simulink model "3R_PD_Regulation_Control"  (R2026a)
settings: Solver=VariableStepAuto
undefined symbols (not defined in the file): X, Y, Z
libraries: nesl_utility x37, sm_lib x29
settings Model: Creator=Bosey  LastModifiedBy=Bosey

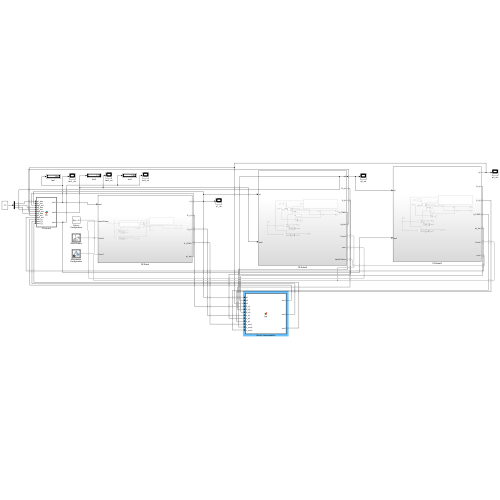
[thumbnail: Simulink's stored preview of the top-level diagram]
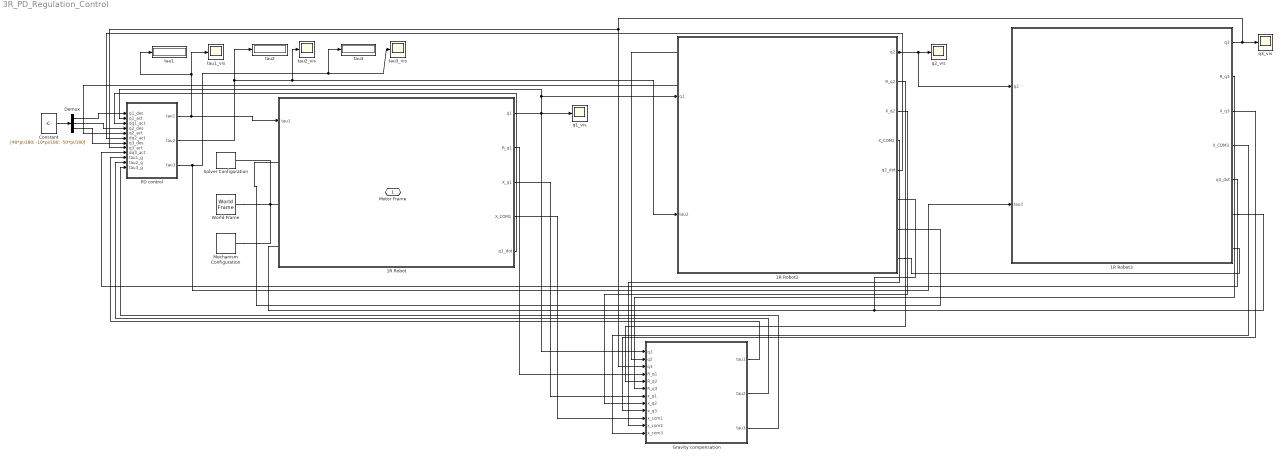
== system 3R_PD_Regulation_Control ==
  1R Robot : Subsystem
  1R Robot2 : Subsystem
  1R Robot3 : Subsystem
  Constant : Constant  Value=[40*pi/180; -10*pi/180; -50*pi/180]
  Demux : Demux  Outputs=3
  Gravity compensation : MATLAB Function  TreatAsAtomicUnit=on
  Mechanism Configuration : sm_lib/Utilities/Mechanism Configuration  UniformGravity=Constant  GravityVector=[0 0 -9.80665]  GravityVectorUnits=m/s^2  LinearizationDelta=0.001  JointModeTransitionNonlinearIterations=2
  PD control : MATLAB Function  TreatAsAtomicUnit=on
  Solver Configuration : nesl_utility/Solver Configuration  PhysicalDomain=network_engine_domain  SubClassName=solver  LeftPortType=input  RightPortType=generic  Tones=[]  Harmonics=[]  SimulateNoise=off  Profile=off  UseLocalSampling=off  EnableSwitchedLinearOptims=on  FrequencyDomain=off  UseCCode=off  RelTol=0.001  AbsTol=1e-06  MinStep=1e-09  ToWorkspace=off  RevertToSquareIcSolve=off  NumHomotopyIterations=100  PhasorMode=off  PhasorModeNumHarmonics=1  ConsistencySolver=NEWTON_XTOL_AFTER_FTOL  CanonicalOrdering=UNORDERED  OptimizeIntermediates=UNOPTIMIZED  IndexReductionMethod=DerivativeReplacement  DoDC=off  ResidualTolerance=1e-09  ConsistencyTolSource=GLOBAL  ConsistencyAbsTol=0.001  ConsistencyRelTol=0.001  ConsistencyTolFactor=0.001  UseLocalSolver=off  LocalSolverChoice=NE_BACKWARD_EULER_ADVANCER  ResolveIndetEquations=on  FunctionEvalNumThread=1  LocalSolverSampleTime=0.001  DoFixedCost=off  MaxNonlinIter=3  MaxModeIter=2  ComputeImpulses=off  ImpulseIterations=2  LinearAlgebra=Sparse  LinearAlgebraNumThread=0  EquationFormulation=NE_TIME_EF  DelaysMemoryBudget=1024  AutomaticFiltering=on  FilteringTimeConstant=0.001  PartitionStorageMethod=AS_NEEDED  PartitionMemoryBudget=1024  PartitionMethod=FAST  MultibodyUseLocalSolver=off  MultibodyLocalSolverChoice=ODE1  MultibodyLocalSolverSampleTime=0.001
  World Frame : sm_lib/Frames and Transforms/World Frame
  q1_vis : Scope
      settings: ActiveDisplayYMinimum=0.2274863959797675  ActiveDisplayYMaximum=1.3862172206154479
  q2_vis : Scope
      settings: ActiveDisplayYMinimum=-0.21838931601721817  ActiveDisplayYMaximum=0.20349654350607727  DataLoggingVariableName=ScopeData4
  q3_vis : Scope
      settings: ActiveDisplayYMinimum=-0.90239032801862251  ActiveDisplayYMaximum=-0.64728032168659821  DataLoggingVariableName=ScopeData11
  tau1 : Display
  tau1_vis : Scope
      settings: ActiveDisplayYMinimum=-1  ActiveDisplayYMaximum=1  DataLoggingVariableName=ScopeData8
  tau2 : Display
  tau2_vis : Scope
      settings: DataLoggingVariableName=ScopeData9
  tau3 : Display
  tau3_vis : Scope
      settings: DataLoggingVariableName=ScopeData10
  Motor Frame : PMIOPort  Side=Left
  wires:
  1R Robot2/1(q2) -> Gravity compensation/2(q2), PD control/5(q2_act), 1R Robot3/1(q2), q2_vis/1
  1R Robot/1(q1) -> Gravity compensation/1(q1), PD control/2(q1_act), 1R Robot2/1(q1), q1_vis/1
  1R Robot/3(X_q1) -> Gravity compensation/7(x_q1)
  1R Robot2/3(X_q2) -> Gravity compensation/8(x_q2)
  1R Robot3/4(X_COM3) -> Gravity compensation/12(x_com3)
  1R Robot3/3(X_q3) -> Gravity compensation/9(x_q3)
  1R Robot2/4(X_COM2) -> Gravity compensation/11(x_com2)
  1R Robot3/1(q3) -> q3_vis/1, PD control/8(q3_act), Gravity compensation/3(q3)
  1R Robot/4(X_COM1) -> Gravity compensation/10(x_com1)
  PD control/1(tau1) -> tau1_vis/1, tau1/1, 1R Robot/1(tau1)
  PD control/2(tau2) -> tau2/1, 1R Robot2/2(tau2), tau2_vis/1
  PD control/3(tau3) -> tau3_vis/1, tau3/1, 1R Robot3/2(tau3)
  1R Robot/5(q1_dot) -> PD control/3(dq1_act)
  1R Robot2/5(q2_dot) -> PD control/6(dq2_act)
  1R Robot3/5(q3_dot) -> PD control/9(dq3_act)
  1R Robot/2(R_q1) -> Gravity compensation/4(R_q1)
  1R Robot2/2(R_q2) -> Gravity compensation/5(R_q2)
  Gravity compensation/1(tau1) -> PD control/10(tau1_g)
  Gravity compensation/2(tau2) -> PD control/11(tau2_g)
  1R Robot3/2(R_q3) -> Gravity compensation/6(R_q3)
  Gravity compensation/3(tau3) -> PD control/12(tau3_g)
  Constant/1 -> Demux/1
  Demux/1 -> PD control/1(q1_des)
  Demux/2 -> PD control/4(q2_des)
  Demux/3 -> PD control/7(q3_des)
  connections:
  Solver Configuration/RConn1 -- Mechanism Configuration/RConn1 -- World Frame/RConn1 -- 1R Robot/LConn2
  1R Robot2/RConn1 -- 1R Robot/LConn3 -- 1R Robot3/RConn1
  1R Robot/LConn1 -- 1R Robot2/RConn2
  1R Robot2/RConn3 -- 1R Robot3/RConn2

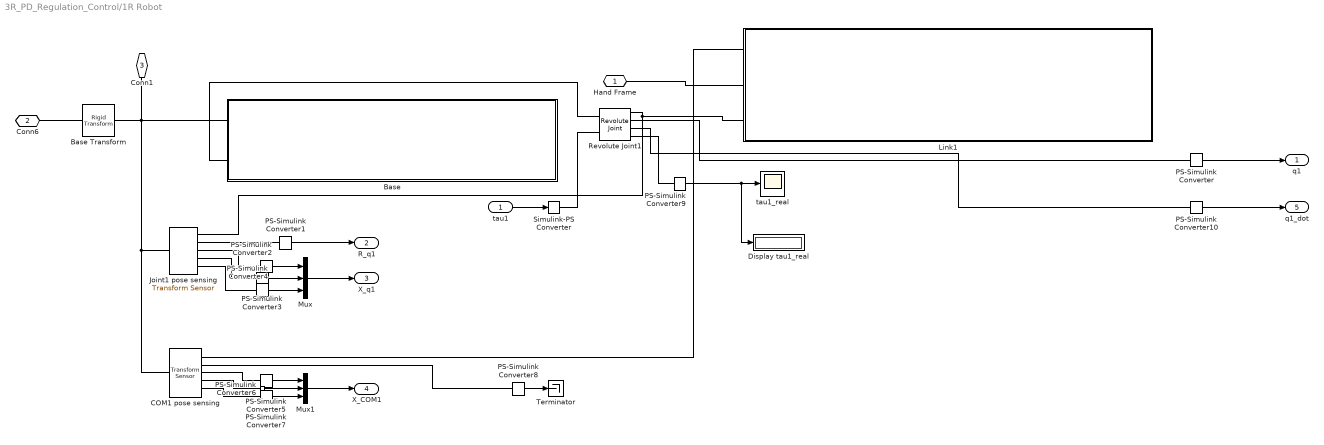
== system 3R_PD_Regulation_Control/1R Robot ==
  tau1 : Inport
  Base : Subsystem
  Base Transform : sm_lib/Frames and Transforms/Rigid Transform  RotationMethod=RotationMatrix  FollAlignAxisA=+Z  BaseAlignAxisA=-Y  FollAlignAxisB=+X  BaseAlignAxisB=+X  RotationStandardAxis=+X  RotationAngle=90  RotationAngleUnits=deg  RotationArbitraryAxis=[0 0 1]  RotationSequenceAxes=BaseAxes  RotationSequence=XYZ  RotationSequenceAngles=[90 0 0]  RotationSequenceAnglesUnits=deg  RotationMatrix=[1 0 0; 0 0 -1; 0 1 0]  Quaternion=[1 0 0 0]  TranslationMethod=None  TranslationCartesianOffset=[0 0 0]  TranslationCartesianOffsetUnits=m  TranslationStandardAxis=+Z  TranslationStandardOffset=0  TranslationStandardOffsetUnits=m  TranslationROffset=0  TranslationROffsetUnits=m  TranslationThetaOffset=0  TranslationThetaOffsetUnits=deg  TranslationZOffset=0  TranslationZOffsetUnits=m
  COM1 pose sensing : sm_lib/Frames and Transforms/Transform Sensor  MeasurementFrame=Base  RotationSequence=XYX  SenseAngle=off  SenseAxis=off  SenseQ=off  SenseR=on  SenseRotationSequence=off  SenseOmegaX=off  SenseOmegaY=off  SenseOmegaZ=off  SenseOmega=off  SenseQDot=off  SenseRDot=off  SenseRotationSequenceDot=off  SenseAlphaX=off  SenseAlphaY=off  SenseAlphaZ=off  SenseAlpha=off  SenseQDDot=off  SenseRDDot=off  SenseX=on  SenseY=on  SenseZ=on  SenseXYZ=off  SenseRad=off  SenseAzim=off  SenseDist=off  SenseInc=off  SenseXDot=off  SenseYDot=off  SenseZDot=off  SenseXYZDot=off  SenseRadDot=off  SenseAzimDot=off  SenseDistDot=off  SenseIncDot=off  SenseXDDot=off  SenseYDDot=off  SenseZDDot=off  SenseXYZDDot=off  SenseRadDDot=off  SenseAzimDDot=off  SenseDistDDot=off  SenseIncDDot=off
  Display tau1_real : Display
  Joint1 pose sensing : sm_lib/Frames and Transforms/Transform Sensor  MeasurementFrame=Base  RotationSequence=XYX  SenseAngle=off  SenseAxis=off  SenseQ=off  SenseR=on  SenseRotationSequence=off  SenseOmegaX=off  SenseOmegaY=off  SenseOmegaZ=off  SenseOmega=off  SenseQDot=off  SenseRDot=off  SenseRotationSequenceDot=off  SenseAlphaX=off  SenseAlphaY=off  SenseAlphaZ=off  SenseAlpha=off  SenseQDDot=off  SenseRDDot=off  SenseX=on  SenseY=on  SenseZ=on  SenseXYZ=off  SenseRad=off  SenseAzim=off  SenseDist=off  SenseInc=off  SenseXDot=off  SenseYDot=off  SenseZDot=off  SenseXYZDot=off  SenseRadDot=off  SenseAzimDot=off  SenseDistDot=off  SenseIncDot=off  SenseXDDot=off  SenseYDDot=off  SenseZDDot=off  SenseXYZDDot=off  SenseRadDDot=off  SenseAzimDDot=off  SenseDistDDot=off  SenseIncDDot=off
  Link1 : Subsystem
  Mux : Mux  Inputs=3
  Mux1 : Mux  Inputs=3
  PS-Simulink Converter{,1..10} (11 alike) : nesl_utility/PS-Simulink Converter  PhysicalDomain=network_engine_domain  SubClassName=ps_output  LeftPortType=input  RightPortType=output  PseudoPeriodic=off  Frequencies=[]  VectorFormat=inherit  Unit=inherit  AffineConversion=off
  Revolute Joint1 : sm_lib/Joints/Revolute Joint  JointMode=Normal  CompositeWrenchDir=FollowerOnBase  CompositeWrenchFrame=BaseFrame  SenseConstraintForce=off  SenseConstraintTorque=off  SenseTotalForce=off  SenseTotalTorque=off  PositionTargetSpecify=on  PositionTargetPriority=High  PositionTargetValue=10  PositionTargetValueUnits=deg  VelocityTargetSpecify=off  VelocityTargetPriority=High  VelocityTargetValue=0  VelocityTargetValueUnits=deg/s  EquilibriumPosition=0  EquilibriumPositionUnits=deg  SpringStiffness=0  SpringStiffnessUnits=N*m/deg  DampingCoefficient=0  DampingCoefficientUnits=N*m/(deg/s)  LowerLimitSpecify=off  LowerLimitBound=-90  LowerLimitBoundUnits=deg  LowerLimitStiffness=1e4  LowerLimitStiffnessUnits=N*m/deg  LowerLimitDamping=10  LowerLimitDampingUnits=N*m/(deg/s)  LowerLimitTransitionRegionWidth=0.1  LowerLimitTransitionRegionWidthUnits=deg  UpperLimitSpecify=off  UpperLimitBound=90  UpperLimitBoundUnits=deg  UpperLimitStiffness=1e4  UpperLimitStiffnessUnits=N*m/deg  UpperLimitDamping=10  UpperLimitDampingUnits=N*m/(deg/s)  UpperLimitTransitionRegionWidth=0.1  UpperLimitTransitionRegionWidthUnits=deg  TorqueActuationMode=InputTorque  MotionActuationMode=ComputedMotion  SensePosition=on  SenseVelocity=on  SenseAcceleration=off  SenseTorqueForce=on  SenseLowerLimitTorqueForce=off  SenseUpperLimitTorqueForce=off
  Simulink-PS Converter : nesl_utility/Simulink-PS Converter  PhysicalDomain=network_engine_domain  SubClassName=ps_input  LeftPortType=input  RightPortType=output  PseudoPeriodic=off  Frequencies=[]  NoiseDistribution=none  NoiseParameters=[]  Unit=1  AffineConversion=off  FilteringAndDerivatives=provide  SimscapeFilterOrder=1  InputFilterTimeConstant=0.001  UdotUserProvided=0
  Terminator : Terminator
  tau1_real : Scope
      settings: ActiveDisplayYMinimum=-1  ActiveDisplayYMaximum=1
  Hand Frame : PMIOPort  Side=Left
  Conn6 : PMIOPort  Port=2  Side=Left
  Conn1 : PMIOPort  Port=3  Side=Left
  q1 : Outport
  R_q1 : Outport  Port=2
  X_q1 : Outport  Port=3
  X_COM1 : Outport  Port=4
  q1_dot : Outport  Port=5
  wires:
  PS-Simulink Converter/1 -> q1/1
  tau1/1 -> Simulink-PS Converter/1
  PS-Simulink Converter1/1 -> R_q1/1
  PS-Simulink Converter2/1 -> Mux/1
  PS-Simulink Converter3/1 -> Mux/2
  PS-Simulink Converter4/1 -> Mux/3
  Mux/1 -> X_q1/1
  PS-Simulink Converter7/1 -> Mux1/3
  PS-Simulink Converter6/1 -> Mux1/2
  PS-Simulink Converter5/1 -> Mux1/1
  Mux1/1 -> X_COM1/1
  PS-Simulink Converter8/1 -> Terminator/1
  PS-Simulink Converter9/1 -> Display tau1_real/1, tau1_real/1
  PS-Simulink Converter10/1 -> q1_dot/1
  connections:
  Conn1/RConn1 -- Base/LConn1 -- Base Transform/RConn1 -- COM1 pose sensing/LConn1 -- Joint1 pose sensing/LConn1
  Base/LConn2 -- Revolute Joint1/LConn1
  Link1/LConn3 -- Joint1 pose sensing/RConn1 -- Revolute Joint1/RConn1
  COM1 pose sensing/RConn1 -- Link1/LConn1
  Revolute Joint1/RConn2 -- PS-Simulink Converter/LConn1
  Simulink-PS Converter/RConn1 -- Revolute Joint1/LConn2
  Joint1 pose sensing/RConn2 -- PS-Simulink Converter1/LConn1
  COM1 pose sensing/RConn3 -- PS-Simulink Converter5/LConn1
  COM1 pose sensing/RConn4 -- PS-Simulink Converter6/LConn1
  COM1 pose sensing/RConn5 -- PS-Simulink Converter7/LConn1
  COM1 pose sensing/RConn2 -- PS-Simulink Converter8/LConn1
  PS-Simulink Converter2/LConn1 -- Joint1 pose sensing/RConn3
  Joint1 pose sensing/RConn5 -- PS-Simulink Converter4/LConn1
  Joint1 pose sensing/RConn4 -- PS-Simulink Converter3/LConn1
  Hand Frame/RConn1 -- Link1/LConn2
  Base Transform/LConn1 -- Conn6/RConn1
  PS-Simulink Converter9/LConn1 -- Revolute Joint1/RConn4
  PS-Simulink Converter10/LConn1 -- Revolute Joint1/RConn3

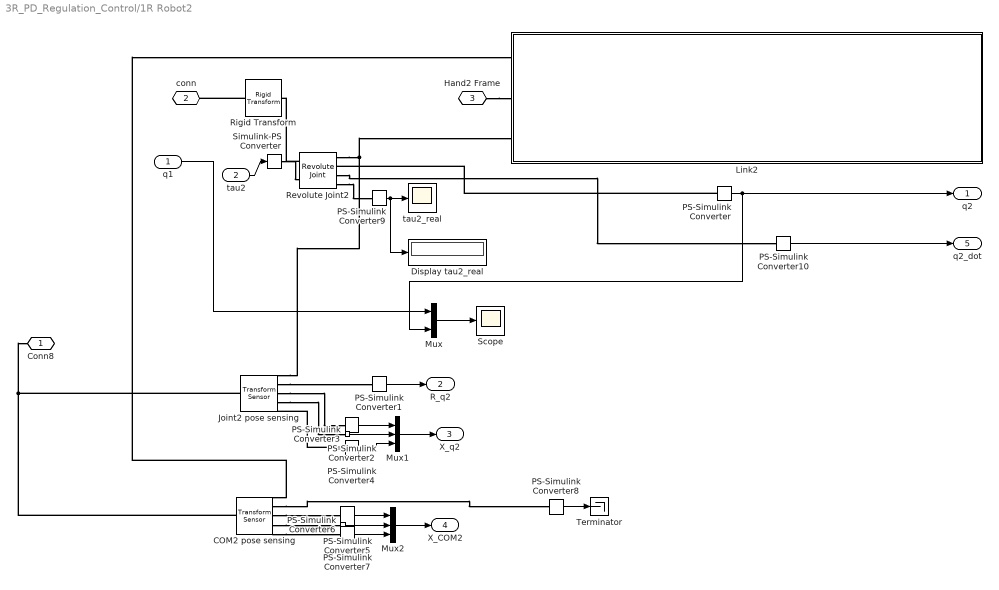
== system 3R_PD_Regulation_Control/1R Robot2 ==
  q1 : Inport
  tau2 : Inport  Port=2
  COM2 pose sensing : sm_lib/Frames and Transforms/Transform Sensor  MeasurementFrame=Base  RotationSequence=XYX  SenseAngle=off  SenseAxis=off  SenseQ=off  SenseR=on  SenseRotationSequence=off  SenseOmegaX=off  SenseOmegaY=off  SenseOmegaZ=off  SenseOmega=off  SenseQDot=off  SenseRDot=off  SenseRotationSequenceDot=off  SenseAlphaX=off  SenseAlphaY=off  SenseAlphaZ=off  SenseAlpha=off  SenseQDDot=off  SenseRDDot=off  SenseX=on  SenseY=on  SenseZ=on  SenseXYZ=off  SenseRad=off  SenseAzim=off  SenseDist=off  SenseInc=off  SenseXDot=off  SenseYDot=off  SenseZDot=off  SenseXYZDot=off  SenseRadDot=off  SenseAzimDot=off  SenseDistDot=off  SenseIncDot=off  SenseXDDot=off  SenseYDDot=off  SenseZDDot=off  SenseXYZDDot=off  SenseRadDDot=off  SenseAzimDDot=off  SenseDistDDot=off  SenseIncDDot=off
  Display tau2_real : Display
  Joint2 pose sensing : sm_lib/Frames and Transforms/Transform Sensor  MeasurementFrame=Base  RotationSequence=XYX  SenseAngle=off  SenseAxis=off  SenseQ=off  SenseR=on  SenseRotationSequence=off  SenseOmegaX=off  SenseOmegaY=off  SenseOmegaZ=off  SenseOmega=off  SenseQDot=off  SenseRDot=off  SenseRotationSequenceDot=off  SenseAlphaX=off  SenseAlphaY=off  SenseAlphaZ=off  SenseAlpha=off  SenseQDDot=off  SenseRDDot=off  SenseX=on  SenseY=on  SenseZ=on  SenseXYZ=off  SenseRad=off  SenseAzim=off  SenseDist=off  SenseInc=off  SenseXDot=off  SenseYDot=off  SenseZDot=off  SenseXYZDot=off  SenseRadDot=off  SenseAzimDot=off  SenseDistDot=off  SenseIncDot=off  SenseXDDot=off  SenseYDDot=off  SenseZDDot=off  SenseXYZDDot=off  SenseRadDDot=off  SenseAzimDDot=off  SenseDistDDot=off  SenseIncDDot=off
  Link2 : Subsystem
  Mux : Mux  Inputs=2
  Mux1 : Mux  Inputs=3
  Mux2 : Mux  Inputs=3
  PS-Simulink Converter{,1..10} (11 alike) : nesl_utility/PS-Simulink Converter  PhysicalDomain=network_engine_domain  SubClassName=ps_output  LeftPortType=input  RightPortType=output  PseudoPeriodic=off  Frequencies=[]  VectorFormat=inherit  Unit=inherit  AffineConversion=off
  Revolute Joint2 : sm_lib/Joints/Revolute Joint  JointMode=Normal  CompositeWrenchDir=FollowerOnBase  CompositeWrenchFrame=BaseFrame  SenseConstraintForce=off  SenseConstraintTorque=off  SenseTotalForce=off  SenseTotalTorque=off  PositionTargetSpecify=on  PositionTargetPriority=High  PositionTargetValue=20  PositionTargetValueUnits=deg  VelocityTargetSpecify=off  VelocityTargetPriority=High  VelocityTargetValue=0  VelocityTargetValueUnits=deg/s  EquilibriumPosition=0  EquilibriumPositionUnits=deg  SpringStiffness=0  SpringStiffnessUnits=N*m/deg  DampingCoefficient=0  DampingCoefficientUnits=N*m/(deg/s)  LowerLimitSpecify=off  LowerLimitBound=-90  LowerLimitBoundUnits=deg  LowerLimitStiffness=1e4  LowerLimitStiffnessUnits=N*m/deg  LowerLimitDamping=10  LowerLimitDampingUnits=N*m/(deg/s)  LowerLimitTransitionRegionWidth=0.1  LowerLimitTransitionRegionWidthUnits=deg  UpperLimitSpecify=off  UpperLimitBound=90  UpperLimitBoundUnits=deg  UpperLimitStiffness=1e4  UpperLimitStiffnessUnits=N*m/deg  UpperLimitDamping=10  UpperLimitDampingUnits=N*m/(deg/s)  UpperLimitTransitionRegionWidth=0.1  UpperLimitTransitionRegionWidthUnits=deg  TorqueActuationMode=InputTorque  MotionActuationMode=ComputedMotion  SensePosition=on  SenseVelocity=on  SenseAcceleration=off  SenseTorqueForce=on  SenseLowerLimitTorqueForce=off  SenseUpperLimitTorqueForce=off
  Rigid Transform : sm_lib/Frames and Transforms/Rigid Transform  RotationMethod=None  FollAlignAxisA=+X  BaseAlignAxisA=+Y  FollAlignAxisB=+Y  BaseAlignAxisB=+Z  RotationStandardAxis=+Z  RotationAngle=90  RotationAngleUnits=deg  RotationArbitraryAxis=[0 0 1]  RotationSequenceAxes=BaseAxes  RotationSequence=XYZ  RotationSequenceAngles=[-90 0 -90]  RotationSequenceAnglesUnits=deg  RotationMatrix=[1 0 0;0 1 0;0 0 1]  Quaternion=[1 0 0 0]  TranslationMethod=None  TranslationCartesianOffset=[0 0 0]  TranslationCartesianOffsetUnits=m  TranslationStandardAxis=+X  TranslationStandardOffset=0.2  TranslationStandardOffsetUnits=m  TranslationROffset=0  TranslationROffsetUnits=m  TranslationThetaOffset=0  TranslationThetaOffsetUnits=deg  TranslationZOffset=0  TranslationZOffsetUnits=m
  Scope : Scope
      settings: ActiveDisplayYMinimum=-3.9555769196396309  ActiveDisplayYMaximum=1.3121731726237904
  Simulink-PS Converter : nesl_utility/Simulink-PS Converter  PhysicalDomain=network_engine_domain  SubClassName=ps_input  LeftPortType=input  RightPortType=output  PseudoPeriodic=off  Frequencies=[]  NoiseDistribution=none  NoiseParameters=[]  Unit=1  AffineConversion=off  FilteringAndDerivatives=provide  SimscapeFilterOrder=1  InputFilterTimeConstant=0.001  UdotUserProvided=0
  Terminator : Terminator
  tau2_real : Scope
      settings: ActiveDisplayYMinimum=-1  ActiveDisplayYMaximum=1  DataLoggingVariableName=ScopeData7
  Conn8 : PMIOPort  Side=Right
  conn : PMIOPort  Port=2  Side=Right
  Hand2 Frame : PMIOPort  Port=3  Side=Right
  q2 : Outport
  R_q2 : Outport  Port=2
  X_q2 : Outport  Port=3
  X_COM2 : Outport  Port=4
  q2_dot : Outport  Port=5
  wires:
  PS-Simulink Converter8/1 -> Terminator/1
  PS-Simulink Converter4/1 -> Mux1/3
  Mux/1 -> Scope/1
  Mux1/1 -> X_q2/1
  PS-Simulink Converter2/1 -> Mux1/1
  PS-Simulink Converter7/1 -> Mux2/3
  PS-Simulink Converter3/1 -> Mux1/2
  PS-Simulink Converter1/1 -> R_q2/1
  PS-Simulink Converter6/1 -> Mux2/2
  Mux2/1 -> X_COM2/1
  PS-Simulink Converter5/1 -> Mux2/1
  q1/1 -> Mux/1
  PS-Simulink Converter9/1 -> Display tau2_real/1, tau2_real/1
  tau2/1 -> Simulink-PS Converter/1
  PS-Simulink Converter/1 -> Mux/2, q2/1
  PS-Simulink Converter10/1 -> q2_dot/1
  connections:
  PS-Simulink Converter4/LConn1 -- Joint2 pose sensing/RConn5
  COM2 pose sensing/RConn1 -- Link2/LConn1
  Revolute Joint2/RConn1 -- Link2/LConn3 -- Joint2 pose sensing/RConn1
  PS-Simulink Converter/LConn1 -- Revolute Joint2/RConn2
  Joint2 pose sensing/RConn3 -- PS-Simulink Converter2/LConn1
  Joint2 pose sensing/LConn1 -- COM2 pose sensing/LConn1 -- Conn8/RConn1
  Joint2 pose sensing/RConn2 -- PS-Simulink Converter1/LConn1
  COM2 pose sensing/RConn5 -- PS-Simulink Converter7/LConn1
  COM2 pose sensing/RConn4 -- PS-Simulink Converter6/LConn1
  COM2 pose sensing/RConn3 -- PS-Simulink Converter5/LConn1
  COM2 pose sensing/RConn2 -- PS-Simulink Converter8/LConn1
  Joint2 pose sensing/RConn4 -- PS-Simulink Converter3/LConn1
  Rigid Transform/LConn1 -- conn/RConn1
  Revolute Joint2/LConn1 -- Rigid Transform/RConn1
  Revolute Joint2/RConn4 -- PS-Simulink Converter9/LConn1
  Revolute Joint2/RConn3 -- PS-Simulink Converter10/LConn1
  Simulink-PS Converter/RConn1 -- Revolute Joint2/LConn2
  Hand2 Frame/RConn1 -- Link2/LConn2

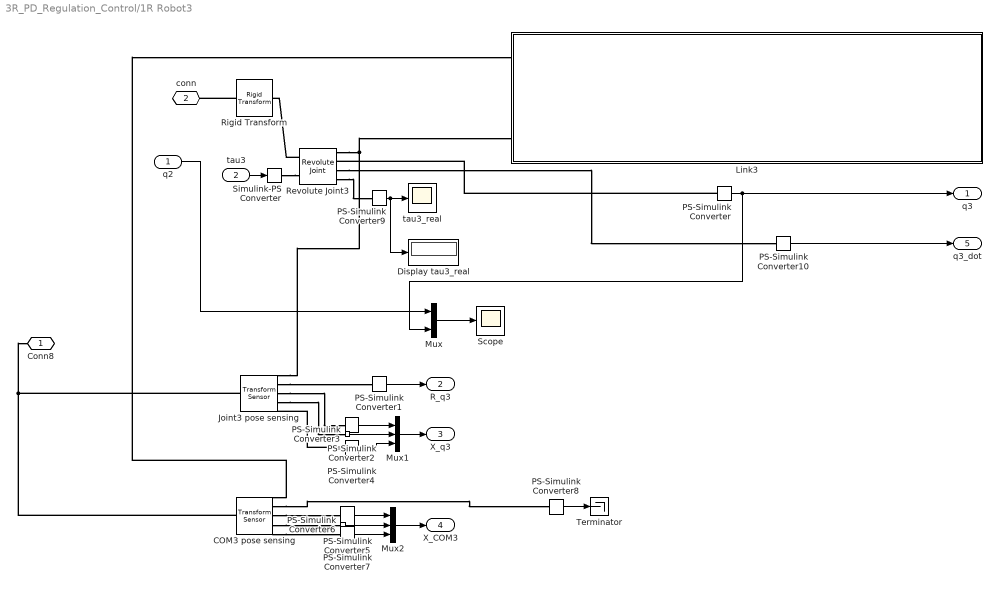
== system 3R_PD_Regulation_Control/1R Robot3 ==
  q2 : Inport
  tau3 : Inport  Port=2
  COM3 pose sensing : sm_lib/Frames and Transforms/Transform Sensor  MeasurementFrame=Base  RotationSequence=XYX  SenseAngle=off  SenseAxis=off  SenseQ=off  SenseR=on  SenseRotationSequence=off  SenseOmegaX=off  SenseOmegaY=off  SenseOmegaZ=off  SenseOmega=off  SenseQDot=off  SenseRDot=off  SenseRotationSequenceDot=off  SenseAlphaX=off  SenseAlphaY=off  SenseAlphaZ=off  SenseAlpha=off  SenseQDDot=off  SenseRDDot=off  SenseX=on  SenseY=on  SenseZ=on  SenseXYZ=off  SenseRad=off  SenseAzim=off  SenseDist=off  SenseInc=off  SenseXDot=off  SenseYDot=off  SenseZDot=off  SenseXYZDot=off  SenseRadDot=off  SenseAzimDot=off  SenseDistDot=off  SenseIncDot=off  SenseXDDot=off  SenseYDDot=off  SenseZDDot=off  SenseXYZDDot=off  SenseRadDDot=off  SenseAzimDDot=off  SenseDistDDot=off  SenseIncDDot=off
  Display tau3_real : Display
  Joint3 pose sensing : sm_lib/Frames and Transforms/Transform Sensor  MeasurementFrame=Base  RotationSequence=XYX  SenseAngle=off  SenseAxis=off  SenseQ=off  SenseR=on  SenseRotationSequence=off  SenseOmegaX=off  SenseOmegaY=off  SenseOmegaZ=off  SenseOmega=off  SenseQDot=off  SenseRDot=off  SenseRotationSequenceDot=off  SenseAlphaX=off  SenseAlphaY=off  SenseAlphaZ=off  SenseAlpha=off  SenseQDDot=off  SenseRDDot=off  SenseX=on  SenseY=on  SenseZ=on  SenseXYZ=off  SenseRad=off  SenseAzim=off  SenseDist=off  SenseInc=off  SenseXDot=off  SenseYDot=off  SenseZDot=off  SenseXYZDot=off  SenseRadDot=off  SenseAzimDot=off  SenseDistDot=off  SenseIncDot=off  SenseXDDot=off  SenseYDDot=off  SenseZDDot=off  SenseXYZDDot=off  SenseRadDDot=off  SenseAzimDDot=off  SenseDistDDot=off  SenseIncDDot=off
  Link3 : Subsystem
  Mux : Mux  Inputs=2
  Mux1 : Mux  Inputs=3
  Mux2 : Mux  Inputs=3
  PS-Simulink Converter{,1..10} (11 alike) : nesl_utility/PS-Simulink Converter  PhysicalDomain=network_engine_domain  SubClassName=ps_output  LeftPortType=input  RightPortType=output  PseudoPeriodic=off  Frequencies=[]  VectorFormat=inherit  Unit=inherit  AffineConversion=off
  Revolute Joint3 : sm_lib/Joints/Revolute Joint  JointMode=Normal  CompositeWrenchDir=FollowerOnBase  CompositeWrenchFrame=BaseFrame  SenseConstraintForce=off  SenseConstraintTorque=off  SenseTotalForce=off  SenseTotalTorque=off  PositionTargetSpecify=on  PositionTargetPriority=High  PositionTargetValue=-30  PositionTargetValueUnits=deg  VelocityTargetSpecify=off  VelocityTargetPriority=High  VelocityTargetValue=0  VelocityTargetValueUnits=deg/s  EquilibriumPosition=0  EquilibriumPositionUnits=deg  SpringStiffness=0  SpringStiffnessUnits=N*m/deg  DampingCoefficient=0  DampingCoefficientUnits=N*m/(deg/s)  LowerLimitSpecify=off  LowerLimitBound=-90  LowerLimitBoundUnits=deg  LowerLimitStiffness=1e4  LowerLimitStiffnessUnits=N*m/deg  LowerLimitDamping=10  LowerLimitDampingUnits=N*m/(deg/s)  LowerLimitTransitionRegionWidth=0.1  LowerLimitTransitionRegionWidthUnits=deg  UpperLimitSpecify=off  UpperLimitBound=90  UpperLimitBoundUnits=deg  UpperLimitStiffness=1e4  UpperLimitStiffnessUnits=N*m/deg  UpperLimitDamping=10  UpperLimitDampingUnits=N*m/(deg/s)  UpperLimitTransitionRegionWidth=0.1  UpperLimitTransitionRegionWidthUnits=deg  TorqueActuationMode=InputTorque  MotionActuationMode=ComputedMotion  SensePosition=on  SenseVelocity=on  SenseAcceleration=off  SenseTorqueForce=on  SenseLowerLimitTorqueForce=off  SenseUpperLimitTorqueForce=off
  Rigid Transform : sm_lib/Frames and Transforms/Rigid Transform  RotationMethod=None  FollAlignAxisA=+X  BaseAlignAxisA=+Y  FollAlignAxisB=+Y  BaseAlignAxisB=+Z  RotationStandardAxis=+Z  RotationAngle=90  RotationAngleUnits=deg  RotationArbitraryAxis=[0 0 1]  RotationSequenceAxes=BaseAxes  RotationSequence=XYZ  RotationSequenceAngles=[-90 0 -90]  RotationSequenceAnglesUnits=deg  RotationMatrix=[1 0 0;0 1 0;0 0 1]  Quaternion=[1 0 0 0]  TranslationMethod=None  TranslationCartesianOffset=[0 0 0]  TranslationCartesianOffsetUnits=m  TranslationStandardAxis=+X  TranslationStandardOffset=0.2  TranslationStandardOffsetUnits=m  TranslationROffset=0  TranslationROffsetUnits=m  TranslationThetaOffset=0  TranslationThetaOffsetUnits=deg  TranslationZOffset=0  TranslationZOffsetUnits=m
  Scope : Scope
      settings: ActiveDisplayYMinimum=-3.9555769196396309  ActiveDisplayYMaximum=1.3121731726237904
  Simulink-PS Converter : nesl_utility/Simulink-PS Converter  PhysicalDomain=network_engine_domain  SubClassName=ps_input  LeftPortType=input  RightPortType=output  PseudoPeriodic=off  Frequencies=[]  NoiseDistribution=none  NoiseParameters=[]  Unit=1  AffineConversion=off  FilteringAndDerivatives=provide  SimscapeFilterOrder=1  InputFilterTimeConstant=0.001  UdotUserProvided=0
  Terminator : Terminator
  tau3_real : Scope
      settings: ActiveDisplayYMinimum=0.20752725828747631  ActiveDisplayYMaximum=1.0145136066212581  DataLoggingVariableName=ScopeData7
  Conn8 : PMIOPort  Side=Right
  conn : PMIOPort  Port=2  Side=Right
  q3 : Outport
  R_q3 : Outport  Port=2
  X_q3 : Outport  Port=3
  X_COM3 : Outport  Port=4
  q3_dot : Outport  Port=5
  wires:
  PS-Simulink Converter8/1 -> Terminator/1
  PS-Simulink Converter4/1 -> Mux1/3
  Mux/1 -> Scope/1
  Mux1/1 -> X_q3/1
  PS-Simulink Converter2/1 -> Mux1/1
  PS-Simulink Converter7/1 -> Mux2/3
  PS-Simulink Converter3/1 -> Mux1/2
  PS-Simulink Converter1/1 -> R_q3/1
  PS-Simulink Converter6/1 -> Mux2/2
  Mux2/1 -> X_COM3/1
  PS-Simulink Converter5/1 -> Mux2/1
  q2/1 -> Mux/1
  PS-Simulink Converter9/1 -> Display tau3_real/1, tau3_real/1
  tau3/1 -> Simulink-PS Converter/1
  PS-Simulink Converter/1 -> Mux/2, q3/1
  PS-Simulink Converter10/1 -> q3_dot/1
  connections:
  PS-Simulink Converter4/LConn1 -- Joint3 pose sensing/RConn5
  COM3 pose sensing/RConn1 -- Link3/LConn1
  Revolute Joint3/RConn1 -- Link3/LConn3 -- Joint3 pose sensing/RConn1
  PS-Simulink Converter/LConn1 -- Revolute Joint3/RConn2
  Joint3 pose sensing/RConn3 -- PS-Simulink Converter2/LConn1
  Joint3 pose sensing/LConn1 -- COM3 pose sensing/LConn1 -- Conn8/RConn1
  Joint3 pose sensing/RConn2 -- PS-Simulink Converter1/LConn1
  COM3 pose sensing/RConn5 -- PS-Simulink Converter7/LConn1
  COM3 pose sensing/RConn4 -- PS-Simulink Converter6/LConn1
  COM3 pose sensing/RConn3 -- PS-Simulink Converter5/LConn1
  COM3 pose sensing/RConn2 -- PS-Simulink Converter8/LConn1
  Joint3 pose sensing/RConn4 -- PS-Simulink Converter3/LConn1
  Rigid Transform/LConn1 -- conn/RConn1
  Revolute Joint3/LConn1 -- Rigid Transform/RConn1
  Revolute Joint3/RConn4 -- PS-Simulink Converter9/LConn1
  Revolute Joint3/RConn3 -- PS-Simulink Converter10/LConn1
  Simulink-PS Converter/RConn1 -- Revolute Joint3/LConn2

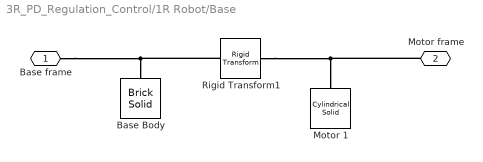
== system 3R_PD_Regulation_Control/1R Robot/Base ==
  "Base Body " : sm_lib/Body Elements/Brick Solid  BrickDimensions=[0.2 0.2 0.02]  BrickDimensionsUnits=m  ExportEntireGeometry=off  InertiaType=CalculateFromGeometry  BasedOnType=Mass  Density=1000  DensityUnits=kg/m^3  Mass=0  MassUnits=kg  CenterOfMass=[0 0 0]  CenterOfMassUnits=m  MomentsOfInertia=[1 1 1]  MomentsOfInertiaUnits=kg*m^2  ProductsOfInertia=[0 0 0]  ProductsOfInertiaUnits=kg*m^2  GraphicType=FromGeometry  MarkerShape=Sphere  MarkerSize=10  GraphicVisPropType=SimpleVisualProperties  GraphicDiffuseColor=[0.502 0.502 0.502]  GraphicOpacity=1.0  GraphicSpecularColor=[0.5 0.5 0.5 1.0]  GraphicAmbientColor=[0.15 0.15 0.15 1.0]  GraphicEmissiveColor=[0.0 0.0 0.0 1.0]  GraphicShininess=75  DoExposeReferenceFrame=on  SerializedFrames=<Frames/>
  Motor 1 : sm_lib/Body Elements/Cylindrical Solid  CylinderRadius=0.02  CylinderRadiusUnits=m  CylinderLength=0.04  CylinderLengthUnits=m  ExportEntireGeometry=off  InertiaType=CalculateFromGeometry  BasedOnType=Mass  Density=1000  DensityUnits=kg/m^3  Mass=0  MassUnits=kg  CenterOfMass=[0 0 0]  CenterOfMassUnits=m  MomentsOfInertia=[1 1 1]  MomentsOfInertiaUnits=kg*m^2  ProductsOfInertia=[0 0 0]  ProductsOfInertiaUnits=kg*m^2  GraphicType=FromGeometry  MarkerShape=Sphere  MarkerSize=10  GraphicVisPropType=SimpleVisualProperties  GraphicDiffuseColor=[0 0 0]  GraphicOpacity=1  GraphicSpecularColor=[0.5 0.5 0.5 1.0]  GraphicAmbientColor=[0.15 0.15 0.15 1.0]  GraphicEmissiveColor=[0.0 0.0 0.0 1.0]  GraphicShininess=75  DoExposeReferenceFrame=on  SerializedFrames=<Frames/>
  Rigid Transform1 : sm_lib/Frames and Transforms/Rigid Transform  RotationMethod=None  FollAlignAxisA=+X  BaseAlignAxisA=+Y  FollAlignAxisB=+Y  BaseAlignAxisB=+Z  RotationStandardAxis=+Z  RotationAngle=0  RotationAngleUnits=deg  RotationArbitraryAxis=[0 0 1]  RotationSequenceAxes=FollowerAxes  RotationSequence=XYX  RotationSequenceAngles=[0 0 0]  RotationSequenceAnglesUnits=deg  RotationMatrix=[1 0 0;0 1 0;0 0 1]  Quaternion=[1 0 0 0]  TranslationMethod=StandardAxis  TranslationCartesianOffset=[0 0 2]  TranslationCartesianOffsetUnits=m  TranslationStandardAxis=+Z  TranslationStandardOffset=0.02  TranslationStandardOffsetUnits=m  TranslationROffset=0  TranslationROffsetUnits=m  TranslationThetaOffset=0  TranslationThetaOffsetUnits=deg  TranslationZOffset=0  TranslationZOffsetUnits=m
  Base frame : PMIOPort  Side=Left
  Motor frame : PMIOPort  Port=2  Side=Left
  connections:
  Rigid Transform1/RConn1 -- Motor frame/RConn1 -- Motor 1/RConn1
  Base frame/RConn1 -- Rigid Transform1/LConn1 -- "Base Body "/RConn1

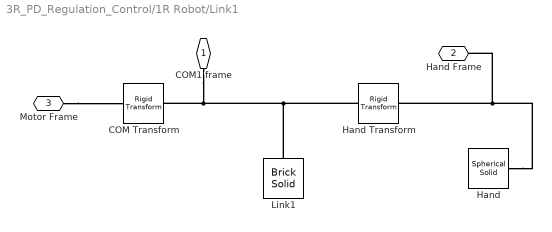
== system 3R_PD_Regulation_Control/1R Robot/Link1 ==
  COM Transform : sm_lib/Frames and Transforms/Rigid Transform  RotationMethod=None  FollAlignAxisA=+X  BaseAlignAxisA=+Y  FollAlignAxisB=+Y  BaseAlignAxisB=+Z  RotationStandardAxis=+Z  RotationAngle=0  RotationAngleUnits=deg  RotationArbitraryAxis=[0 0 1]  RotationSequenceAxes=FollowerAxes  RotationSequence=XYX  RotationSequenceAngles=[0 0 0]  RotationSequenceAnglesUnits=deg  RotationMatrix=[1 0 0;0 1 0;0 0 1]  Quaternion=[1 0 0 0]  TranslationMethod=StandardAxis  TranslationCartesianOffset=[0 0 0]  TranslationCartesianOffsetUnits=m  TranslationStandardAxis=+X  TranslationStandardOffset=0.1  TranslationStandardOffsetUnits=m  TranslationROffset=0  TranslationROffsetUnits=m  TranslationThetaOffset=0  TranslationThetaOffsetUnits=deg  TranslationZOffset=0  TranslationZOffsetUnits=m
  Hand Transform : sm_lib/Frames and Transforms/Rigid Transform  RotationMethod=None  FollAlignAxisA=+Z  BaseAlignAxisA=+X  FollAlignAxisB=+Y  BaseAlignAxisB=-Z  RotationStandardAxis=+Z  RotationAngle=0  RotationAngleUnits=deg  RotationArbitraryAxis=[0 0 1]  RotationSequenceAxes=FollowerAxes  RotationSequence=XYX  RotationSequenceAngles=[0 0 0]  RotationSequenceAnglesUnits=deg  RotationMatrix=[1 0 0;0 1 0;0 0 1]  Quaternion=[1 0 0 0]  TranslationMethod=StandardAxis  TranslationCartesianOffset=[0 0 0]  TranslationCartesianOffsetUnits=m  TranslationStandardAxis=+X  TranslationStandardOffset=0.1  TranslationStandardOffsetUnits=m  TranslationROffset=0  TranslationROffsetUnits=m  TranslationThetaOffset=0  TranslationThetaOffsetUnits=deg  TranslationZOffset=0  TranslationZOffsetUnits=m
  "Hand " : sm_lib/Body Elements/Spherical Solid  SphereRadius=0.01  SphereRadiusUnits=m  ExportEntireGeometry=off  InertiaType=CalculateFromGeometry  BasedOnType=Mass  Density=1000  DensityUnits=kg/m^3  Mass=0  MassUnits=kg  CenterOfMass=[0 0 0]  CenterOfMassUnits=m  MomentsOfInertia=[1 1 1]  MomentsOfInertiaUnits=kg*m^2  ProductsOfInertia=[0 0 0]  ProductsOfInertiaUnits=kg*m^2  GraphicType=FromGeometry  MarkerShape=Sphere  MarkerSize=10  GraphicVisPropType=SimpleVisualProperties  GraphicDiffuseColor=[0.04314 0 0.502]  GraphicOpacity=1  GraphicSpecularColor=[0.5 0.5 0.5 1.0]  GraphicAmbientColor=[0.15 0.15 0.15 1.0]  GraphicEmissiveColor=[0.0 0.0 0.0 1.0]  GraphicShininess=75  DoExposeReferenceFrame=on  SerializedFrames=<Frames/>
  Link1 : sm_lib/Body Elements/Brick Solid  BrickDimensions=[0.2 0.01 0.01]  BrickDimensionsUnits=m  ExportEntireGeometry=off  InertiaType=CalculateFromGeometry  BasedOnType=Mass  Density=1000  DensityUnits=kg/m^3  Mass=2.5  MassUnits=kg  CenterOfMass=[0 0 0]  CenterOfMassUnits=m  MomentsOfInertia=[1 1 1]  MomentsOfInertiaUnits=kg*m^2  ProductsOfInertia=[0 0 0]  ProductsOfInertiaUnits=kg*m^2  GraphicType=FromGeometry  MarkerShape=Sphere  MarkerSize=10  GraphicVisPropType=SimpleVisualProperties  GraphicDiffuseColor=[0.6667 0 0]  GraphicOpacity=1  GraphicSpecularColor=[0.5 0.5 0.5 1.0]  GraphicAmbientColor=[0.15 0.15 0.15 1.0]  GraphicEmissiveColor=[0.0 0.0 0.0 1.0]  GraphicShininess=75  DoExposeReferenceFrame=on  SerializedFrames=<Frames/>
  COM1 frame : PMIOPort  Side=Left
  Hand Frame : PMIOPort  Port=2  Side=Left
  Motor Frame : PMIOPort  Port=3  Side=Left
  connections:
  "Hand "/RConn1 -- Hand Frame/RConn1 -- Hand Transform/RConn1
  Link1/RConn1 -- Hand Transform/LConn1 -- COM Transform/RConn1 -- COM1 frame/RConn1
  Motor Frame/RConn1 -- COM Transform/LConn1

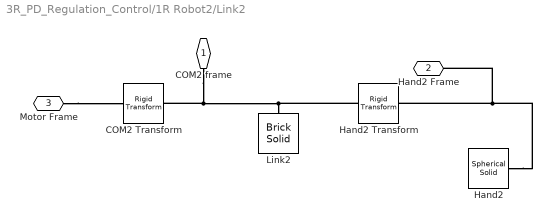
== system 3R_PD_Regulation_Control/1R Robot2/Link2 ==
  COM2 Transform : sm_lib/Frames and Transforms/Rigid Transform  RotationMethod=None  FollAlignAxisA=+X  BaseAlignAxisA=+Y  FollAlignAxisB=+Y  BaseAlignAxisB=+Z  RotationStandardAxis=+Z  RotationAngle=-90  RotationAngleUnits=deg  RotationArbitraryAxis=[0 0 1]  RotationSequenceAxes=FollowerAxes  RotationSequence=XYX  RotationSequenceAngles=[0 0 0]  RotationSequenceAnglesUnits=deg  RotationMatrix=[1 0 0;0 1 0;0 0 1]  Quaternion=[1 0 0 0]  TranslationMethod=StandardAxis  TranslationCartesianOffset=[0 0 0]  TranslationCartesianOffsetUnits=m  TranslationStandardAxis=+X  TranslationStandardOffset=0.1  TranslationStandardOffsetUnits=m  TranslationROffset=0  TranslationROffsetUnits=m  TranslationThetaOffset=0  TranslationThetaOffsetUnits=deg  TranslationZOffset=0  TranslationZOffsetUnits=m
  Hand2 Transform : sm_lib/Frames and Transforms/Rigid Transform  RotationMethod=None  FollAlignAxisA=+X  BaseAlignAxisA=+Y  FollAlignAxisB=+Y  BaseAlignAxisB=+Z  RotationStandardAxis=+Z  RotationAngle=0  RotationAngleUnits=deg  RotationArbitraryAxis=[0 0 1]  RotationSequenceAxes=FollowerAxes  RotationSequence=XYX  RotationSequenceAngles=[0 0 0]  RotationSequenceAnglesUnits=deg  RotationMatrix=[1 0 0;0 1 0;0 0 1]  Quaternion=[1 0 0 0]  TranslationMethod=StandardAxis  TranslationCartesianOffset=[0 0 0]  TranslationCartesianOffsetUnits=m  TranslationStandardAxis=+X  TranslationStandardOffset=0.1  TranslationStandardOffsetUnits=m  TranslationROffset=0  TranslationROffsetUnits=m  TranslationThetaOffset=0  TranslationThetaOffsetUnits=deg  TranslationZOffset=0  TranslationZOffsetUnits=m
  "Hand2 " : sm_lib/Body Elements/Spherical Solid  SphereRadius=0.01  SphereRadiusUnits=m  ExportEntireGeometry=off  InertiaType=CalculateFromGeometry  BasedOnType=Mass  Density=1000  DensityUnits=kg/m^3  Mass=0  MassUnits=kg  CenterOfMass=[0 0 0]  CenterOfMassUnits=m  MomentsOfInertia=[1 1 1]  MomentsOfInertiaUnits=kg*m^2  ProductsOfInertia=[0 0 0]  ProductsOfInertiaUnits=kg*m^2  GraphicType=FromGeometry  MarkerShape=Sphere  MarkerSize=10  GraphicVisPropType=SimpleVisualProperties  GraphicDiffuseColor=[0.04314 0 0.502]  GraphicOpacity=1  GraphicSpecularColor=[0.5 0.5 0.5 1.0]  GraphicAmbientColor=[0.15 0.15 0.15 1.0]  GraphicEmissiveColor=[0.0 0.0 0.0 1.0]  GraphicShininess=75  DoExposeReferenceFrame=on  SerializedFrames=<Frames/>
  Link2 : sm_lib/Body Elements/Brick Solid  BrickDimensions=[0.2 0.01 0.01]  BrickDimensionsUnits=m  ExportEntireGeometry=off  InertiaType=CalculateFromGeometry  BasedOnType=Mass  Density=1000  DensityUnits=kg/m^3  Mass=4.5  MassUnits=kg  CenterOfMass=[0 0 0]  CenterOfMassUnits=m  MomentsOfInertia=[1 1 1]  MomentsOfInertiaUnits=kg*m^2  ProductsOfInertia=[0 0 0]  ProductsOfInertiaUnits=kg*m^2  GraphicType=FromGeometry  MarkerShape=Sphere  MarkerSize=10  GraphicVisPropType=SimpleVisualProperties  GraphicDiffuseColor=[0.6667 0 0]  GraphicOpacity=1  GraphicSpecularColor=[0.5 0.5 0.5 1.0]  GraphicAmbientColor=[0.15 0.15 0.15 1.0]  GraphicEmissiveColor=[0.0 0.0 0.0 1.0]  GraphicShininess=75  DoExposeReferenceFrame=on  SerializedFrames=<Frames/>
  COM2 frame : PMIOPort  Side=Left
  Hand2 Frame : PMIOPort  Port=2  Side=Left
  Motor Frame : PMIOPort  Port=3  Side=Left
  connections:
  Hand2 Transform/RConn1 -- "Hand2 "/RConn1 -- Hand2 Frame/RConn1
  Hand2 Transform/LConn1 -- Link2/RConn1 -- COM2 Transform/RConn1 -- COM2 frame/RConn1
  Motor Frame/RConn1 -- COM2 Transform/LConn1

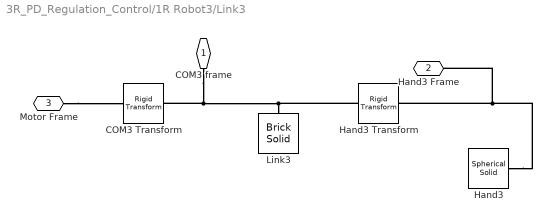
== system 3R_PD_Regulation_Control/1R Robot3/Link3 ==
  COM3 Transform : sm_lib/Frames and Transforms/Rigid Transform  RotationMethod=None  FollAlignAxisA=+X  BaseAlignAxisA=+Y  FollAlignAxisB=+Y  BaseAlignAxisB=+Z  RotationStandardAxis=+Z  RotationAngle=-90  RotationAngleUnits=deg  RotationArbitraryAxis=[0 0 1]  RotationSequenceAxes=FollowerAxes  RotationSequence=XYX  RotationSequenceAngles=[0 0 0]  RotationSequenceAnglesUnits=deg  RotationMatrix=[1 0 0;0 1 0;0 0 1]  Quaternion=[1 0 0 0]  TranslationMethod=StandardAxis  TranslationCartesianOffset=[0 0 0]  TranslationCartesianOffsetUnits=m  TranslationStandardAxis=+X  TranslationStandardOffset=0.1  TranslationStandardOffsetUnits=m  TranslationROffset=0  TranslationROffsetUnits=m  TranslationThetaOffset=0  TranslationThetaOffsetUnits=deg  TranslationZOffset=0  TranslationZOffsetUnits=m
  Hand3 Transform : sm_lib/Frames and Transforms/Rigid Transform  RotationMethod=None  FollAlignAxisA=+X  BaseAlignAxisA=+Y  FollAlignAxisB=+Y  BaseAlignAxisB=+Z  RotationStandardAxis=+Z  RotationAngle=0  RotationAngleUnits=deg  RotationArbitraryAxis=[0 0 1]  RotationSequenceAxes=FollowerAxes  RotationSequence=XYX  RotationSequenceAngles=[0 0 0]  RotationSequenceAnglesUnits=deg  RotationMatrix=[1 0 0;0 1 0;0 0 1]  Quaternion=[1 0 0 0]  TranslationMethod=StandardAxis  TranslationCartesianOffset=[0 0 0]  TranslationCartesianOffsetUnits=m  TranslationStandardAxis=+X  TranslationStandardOffset=0.1  TranslationStandardOffsetUnits=m  TranslationROffset=0  TranslationROffsetUnits=m  TranslationThetaOffset=0  TranslationThetaOffsetUnits=deg  TranslationZOffset=0  TranslationZOffsetUnits=m
  "Hand3 " : sm_lib/Body Elements/Spherical Solid  SphereRadius=0.01  SphereRadiusUnits=m  ExportEntireGeometry=off  InertiaType=CalculateFromGeometry  BasedOnType=Mass  Density=1000  DensityUnits=kg/m^3  Mass=0  MassUnits=kg  CenterOfMass=[0 0 0]  CenterOfMassUnits=m  MomentsOfInertia=[1 1 1]  MomentsOfInertiaUnits=kg*m^2  ProductsOfInertia=[0 0 0]  ProductsOfInertiaUnits=kg*m^2  GraphicType=FromGeometry  MarkerShape=Sphere  MarkerSize=10  GraphicVisPropType=SimpleVisualProperties  GraphicDiffuseColor=[0.04314 0 0.502]  GraphicOpacity=1  GraphicSpecularColor=[0.5 0.5 0.5 1.0]  GraphicAmbientColor=[0.15 0.15 0.15 1.0]  GraphicEmissiveColor=[0.0 0.0 0.0 1.0]  GraphicShininess=75  DoExposeReferenceFrame=on  SerializedFrames=<Frames/>
  Link3 : sm_lib/Body Elements/Brick Solid  BrickDimensions=[0.2 0.01 0.01]  BrickDimensionsUnits=m  ExportEntireGeometry=off  InertiaType=CalculateFromGeometry  BasedOnType=Mass  Density=1000  DensityUnits=kg/m^3  Mass=1.5  MassUnits=kg  CenterOfMass=[0 0 0]  CenterOfMassUnits=m  MomentsOfInertia=[1 1 1]  MomentsOfInertiaUnits=kg*m^2  ProductsOfInertia=[0 0 0]  ProductsOfInertiaUnits=kg*m^2  GraphicType=FromGeometry  MarkerShape=Sphere  MarkerSize=10  GraphicVisPropType=SimpleVisualProperties  GraphicDiffuseColor=[0.6667 0 0]  GraphicOpacity=1  GraphicSpecularColor=[0.5 0.5 0.5 1.0]  GraphicAmbientColor=[0.15 0.15 0.15 1.0]  GraphicEmissiveColor=[0.0 0.0 0.0 1.0]  GraphicShininess=75  DoExposeReferenceFrame=on  SerializedFrames=<Frames/>
  COM3 frame : PMIOPort  Side=Left
  Hand3 Frame : PMIOPort  Port=2  Side=Left
  Motor Frame : PMIOPort  Port=3  Side=Left
  connections:
  Hand3 Transform/RConn1 -- "Hand3 "/RConn1 -- Hand3 Frame/RConn1
  Hand3 Transform/LConn1 -- Link3/RConn1 -- COM3 Transform/RConn1 -- COM3 frame/RConn1
  Motor Frame/RConn1 -- COM3 Transform/LConn1

== matlab function 3R_PD_Regulation_Control/Gravity compensation ==
  data: q1 input; tau1 output; q2 input; q3 input; R_q1 input; R_q2 input; R_q3 input; x_q1 input; x_q2 input; x_q3 input; x_com1 input; x_com2 input; tau2 output; x_com3 input; tau3 output
function [tau1, tau2, tau3] = fcn(q1, q2, q3, R_q1, R_q2, R_q3, x_q1, x_q2, x_q3, x_com1, x_com2, x_com3)
    % Gravity vector
    g_vector = [0; -9.80665; 0]; 
    
    % Masses
    m1 = 2.5;
    m2 = 4.5;
    m3 = 1.5;
    
    % Current rotation axes (Z-axes) from Rotation Matrices
    z1 = R_q1(:, 3); 
    z2 = R_q2(:, 3);
    z3 = R_q3(:, 3);
    
    % Lever Arms (r)
    % Vectors to COM 1
    r11 = x_com1 - x_q1;   
    
    % Vectors to COM 2
    r21 = x_com2 - x_q1;   
    r22 = x_com2 - x_q2;   
    
    % Vectors to COM 3
    r31 = x_com3 - x_q1;   % From Joint 1 to COM 3
    r32 = x_com3 - x_q2;   % From Joint 2 to COM 3
    r33 = x_com3 - x_q3;   % From Joint 3 to COM 3
    
    % Geometric Jacobians (J = z x r) expanded to 3 columns
    % Jacobian for Link 1 COM
    J_com1 = [cross(z1, r11), [0; 0; 0], [0; 0; 0]];
    
    % Jacobian for Link 2 COM
    J_com2 = [cross(z1, r21), cross(z2, r22), [0; 0; 0]];
    
    % Jacobian for Link 3 COM
    J_com3 = [cross(z1, r31), cross(z2, r32), cross(z3, r33)];
    
    % Static torque from balancing equation (tau = -J^T * F)
    % Calculate Gravity Forces
    F_g1 = m1 * g_vector;
    F_g2 = m2 * g_vector;
    F_g3 = m3 * g_vector;
    
    % The total torque vector 
    tau_total = -(J_com1' * F_g1 + J_com2' * F_g2 + J_com3' * F_g3);
    
    % Map to scalar outputs
    tau1 = tau_total(1);
    tau2 = tau_total(2);
    tau3 = tau_total(3);
end

== matlab function 3R_PD_Regulation_Control/PD control ==
  data: q1_des input; q1_act input; dq1_act input; q2_des input; tau1 output; q2_act input; dq2_act input; q3_des input; q3_act input; dq3_act input; tau2 output; tau1_g input; tau2_g input; tau3_g input; tau3 output
function [tau1, tau2, tau3] = fcn(q1_des , q1_act, dq1_act, q2_des , q2_act, dq2_act, q3_des , q3_act, dq3_act, tau1_g, tau2_g, tau3_g)
    % Define Control Gains 
    Kp = 5; % Proportional gain 
    Kd = 4.5;  % Derivative gain 
    
    % PD Control Law + Gravity Compensation
    tau1 = Kp * (q1_des - q1_act) - Kd * dq1_act + tau1_g;
    tau2 = Kp * (q2_des - q2_act) - Kd * dq2_act + tau2_g;
    tau3 = Kp * (q3_des - q3_act) - Kd * dq3_act + tau3_g;

end
